simulink model "CP_Gammatone_Filter"  (R2019b)
settings: Solver=VariableStepAuto  StartTime=0.0  StopTime=testtime  RelTol=1e-3
InitFcn:
  | CP_Gammatone_Test_Parameters
StopFcn:
  | Verify_CP_Gammatone_Filter
values from neighbouring files (symbols this model uses):
  cordiciterationswb = 52    [CP_Gammatone_Test_Parameters.m]
  delta_phase = -TWOPI*centerfreq*tdres    [CP_Gammatone_Test_Parameters.m]
  Fs = 48e3    (= 48000)    [CP_Gammatone_Test_Parameters.m]
  tauwb = 0.003    [CP_Gammatone_Test_Parameters.m]
  tdres = 1/Fs    (= 2.08333333333e-05)    [CP_Gammatone_Test_Parameters.m]
  wbgain = 40.766    [CP_Gammatone_Test_Parameters.m]
undefined symbols (not defined in the file or in its folder): jsin
libraries: dspsrcs4 x2
settings Model: Creator=mblun  LastModifiedBy=t96f346
settings SFSimCC: CustomCodeUndefinedFunction=UseInterfaceOnly

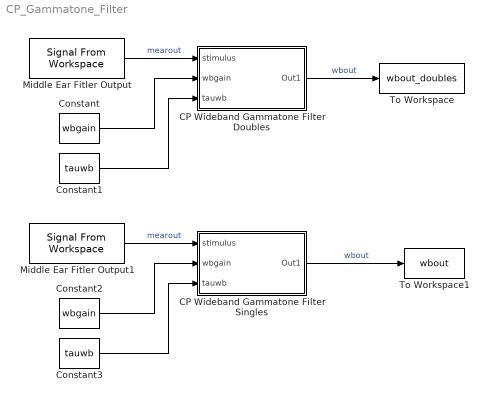
== system CP_Gammatone_Filter ==
  CP Wideband Gammatone Filter Doubles : Subsystem
  CP Wideband Gammatone Filter Singles : Subsystem
  Constant : Constant  Value=wbgain  SampleTime=-1
  Constant1 : Constant  Value=tauwb  SampleTime=-1
  Constant2 : Constant  Value=wbgain  OutDataTypeStr=single  SampleTime=-1
  Constant3 : Constant  Value=tauwb  OutDataTypeStr=single  SampleTime=-1
  Middle Ear Fitler Output : dspsrcs4/Signal From Workspace  X=RxSignal_doubles  Ts=1/Fs  nsamps=1  OutputAfterFinalValue=Setting to zero  ignoreOrWarnInputAndFrameLengths=off  OutputFrames=off
  Middle Ear Fitler Output1 : dspsrcs4/Signal From Workspace  X=RxSignal  Ts=1/Fs  nsamps=1  OutputAfterFinalValue=Setting to zero  ignoreOrWarnInputAndFrameLengths=off  OutputFrames=off
  To Workspace : ToWorkspace  VariableName=wbout_doubles  SampleTime=-1
      settings: Save2DSignal=2-D array (concatenate along first dimension)
  To Workspace1 : ToWorkspace  VariableName=wbout  SampleTime=-1
      settings: Save2DSignal=2-D array (concatenate along first dimension)
  wires:
  Middle Ear Fitler Output/1 -> CP Wideband Gammatone Filter Doubles/1(stimulus)  "mearout"
  CP Wideband Gammatone Filter Doubles/1(Out1) -> To Workspace/1  "wbout"
  Constant/1 -> CP Wideband Gammatone Filter Doubles/2(wbgain)
  Constant1/1 -> CP Wideband Gammatone Filter Doubles/3(tauwb)
  Constant3/1 -> CP Wideband Gammatone Filter Singles/3(tauwb)
  Middle Ear Fitler Output1/1 -> CP Wideband Gammatone Filter Singles/1(stimulus)  "mearout"
  CP Wideband Gammatone Filter Singles/1(Out1) -> To Workspace1/1  "wbout"
  Constant2/1 -> CP Wideband Gammatone Filter Singles/2(wbgain)

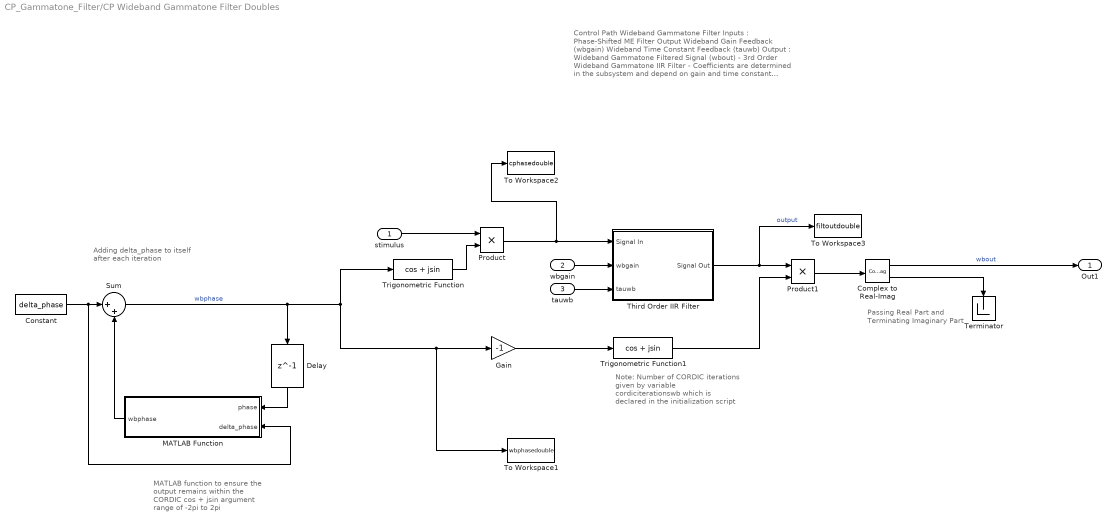
== system CP_Gammatone_Filter/CP Wideband Gammatone Filter Doubles ==
  note: Adding delta_phase to itself after each iteration
  note: Note: Number of CORDIC iterations given by variable cordiciterationswb which is declared in the initialization script
  note: MATLAB function to ensure the output remains within the CORDIC cos + jsin argument range of -2pi to 2pi
  note: Control Path Wideband Gammatone Filter
      |
      | Inputs : Phase-Shifted ME Filter Output
      | Wideband Gain Feedback (wbgain)
      | Wideband Time Constant Feedback (tauwb)
      |
      | Output : Wideband Gammatone Filtered Signal (wbout)
      |
      | - 3rd Order Wideband Gammatone IIR Filter
      |
      | - Coefficients are determined in the subsystem and depend on gain and time constant feedback, set to constants for testing
      |
      | - Implemented w/ Direct Form I Block Structure
  note: Passing Real Part and Terminating Imaginary Part
  stimulus : Inport
  wbgain : Inport  Port=2
  tauwb : Inport  Port=3
  Complex to Real-Imag : ComplexToRealImag
  Constant : Constant  Value=delta_phase  SampleTime=-1
  Delay : Delay  DelayLength=1  InitialCondition=0  UseCircularBuffer=on
  Gain : Gain  Gain=-1
  MATLAB Function : MATLAB Function  TreatAsAtomicUnit=on
  Product : Product
  Product1 : Product
  Sum : Sum  Inputs=|++
  Terminator : Terminator
  Third Order IIR Filter : Subsystem
  To Workspace1 : ToWorkspace  VariableName=wbphasedouble  SampleTime=-1
      settings: Save2DSignal=2-D array (concatenate along first dimension)
  To Workspace2 : ToWorkspace  VariableName=cphasedouble  SampleTime=-1
      settings: Save2DSignal=2-D array (concatenate along first dimension)
  To Workspace3 : ToWorkspace  VariableName=filtoutdouble  SampleTime=-1
      settings: Save2DSignal=2-D array (concatenate along first dimension)
  Trigonometric Function : Trigonometry  Operator=cos + jsin  ApproximationMethod=CORDIC  NumberOfIterations=cordiciterationswb
  Trigonometric Function1 : Trigonometry  Operator=cos + jsin  ApproximationMethod=CORDIC  NumberOfIterations=cordiciterationswb
  Out1 : Outport  VectorParamsAs1DForOutWhenUnconnected=off
  wires:
  wbgain/1 -> Third Order IIR Filter/2(wbgain)
  Gain/1 -> Trigonometric Function1/1
  tauwb/1 -> Third Order IIR Filter/3(tauwb)
  Complex to Real-Imag/2 -> Terminator/1
  Trigonometric Function1/1 -> Product1/2
  Product/1 -> To Workspace2/1, Third Order IIR Filter/1(Signal In)
  Sum/1 -> To Workspace1/1, Gain/1, Trigonometric Function/1, Delay/1  "wbphase"
  Trigonometric Function/1 -> Product/2
  Complex to Real-Imag/1 -> Out1/1  "wbout"
  Constant/1 -> Sum/1, MATLAB Function/2(delta_phase)
  stimulus/1 -> Product/1
  Product1/1 -> Complex to Real-Imag/1
  Third Order IIR Filter/1(Signal Out) -> To Workspace3/1, Product1/1  "output"
  Delay/1 -> MATLAB Function/1(phase)
  MATLAB Function/1(wbphase) -> Sum/2

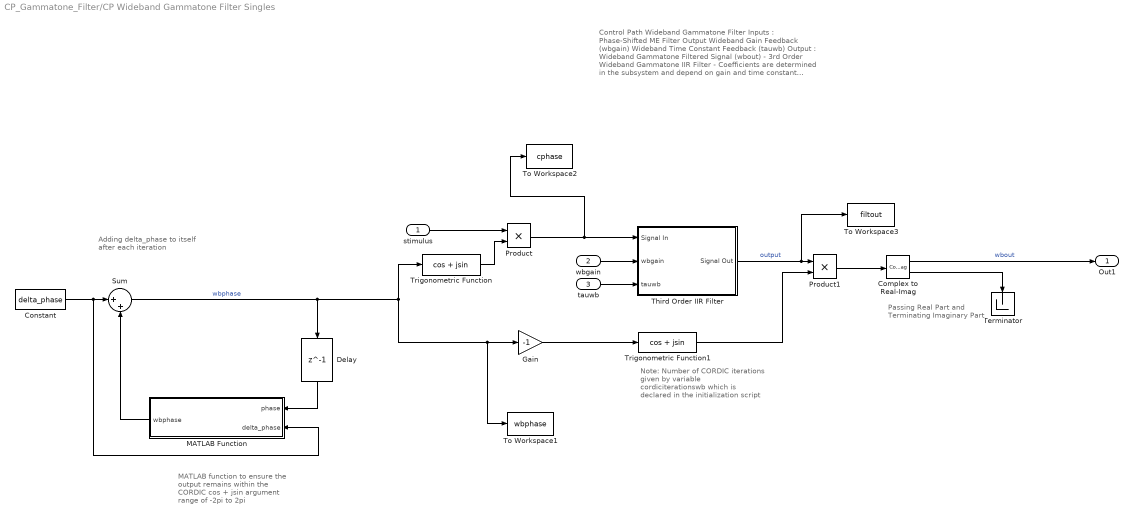
== system CP_Gammatone_Filter/CP Wideband Gammatone Filter Singles ==
  note: Adding delta_phase to itself after each iteration
  note: Note: Number of CORDIC iterations given by variable cordiciterationswb which is declared in the initialization script
  note: MATLAB function to ensure the output remains within the CORDIC cos + jsin argument range of -2pi to 2pi
  note: Control Path Wideband Gammatone Filter
      |
      | Inputs : Phase-Shifted ME Filter Output
      | Wideband Gain Feedback (wbgain)
      | Wideband Time Constant Feedback (tauwb)
      |
      | Output : Wideband Gammatone Filtered Signal (wbout)
      |
      | - 3rd Order Wideband Gammatone IIR Filter
      |
      | - Coefficients are determined in the subsystem and depend on gain and time constant feedback, set to constants for testing
      |
      | - Implemented w/ Direct Form I Block Structure
  note: Passing Real Part and Terminating Imaginary Part
  stimulus : Inport  OutDataTypeStr=single
  wbgain : Inport  Port=2  OutDataTypeStr=single
  tauwb : Inport  Port=3  OutDataTypeStr=single
  Complex to Real-Imag : ComplexToRealImag
  Constant : Constant  Value=delta_phase  OutDataTypeStr=single  SampleTime=-1
  Delay : Delay  DelayLength=1  InitialCondition=0  UseCircularBuffer=on
  Gain : Gain  Gain=-1  OutDataTypeStr=single
  MATLAB Function : MATLAB Function  TreatAsAtomicUnit=on
  Product : Product  OutDataTypeStr=single
  Product1 : Product  OutDataTypeStr=single
  Sum : Sum  Inputs=|++  AccumDataTypeStr=single  OutDataTypeStr=single
  Terminator : Terminator
  Third Order IIR Filter : Subsystem
  To Workspace1 : ToWorkspace  VariableName=wbphase  SampleTime=-1
      settings: Save2DSignal=2-D array (concatenate along first dimension)
  To Workspace2 : ToWorkspace  VariableName=cphase  SampleTime=-1
      settings: Save2DSignal=2-D array (concatenate along first dimension)
  To Workspace3 : ToWorkspace  VariableName=filtout  SampleTime=-1
      settings: Save2DSignal=2-D array (concatenate along first dimension)
  Trigonometric Function : Trigonometry  Operator=cos + jsin  ApproximationMethod=CORDIC  NumberOfIterations=cordiciterationswb
  Trigonometric Function1 : Trigonometry  Operator=cos + jsin  ApproximationMethod=CORDIC  NumberOfIterations=cordiciterationswb
  Out1 : Outport  VectorParamsAs1DForOutWhenUnconnected=off
  wires:
  wbgain/1 -> Third Order IIR Filter/2(wbgain)
  Gain/1 -> Trigonometric Function1/1
  tauwb/1 -> Third Order IIR Filter/3(tauwb)
  Complex to Real-Imag/2 -> Terminator/1
  Trigonometric Function1/1 -> Product1/2
  Product/1 -> To Workspace2/1, Third Order IIR Filter/1(Signal In)
  Sum/1 -> Delay/1, To Workspace1/1, Gain/1, Trigonometric Function/1  "wbphase"
  Trigonometric Function/1 -> Product/2
  Complex to Real-Imag/1 -> Out1/1  "wbout"
  Constant/1 -> Sum/1, MATLAB Function/2(delta_phase)
  stimulus/1 -> Product/1
  Product1/1 -> Complex to Real-Imag/1
  Third Order IIR Filter/1(Signal Out) -> To Workspace3/1, Product1/1  "output"
  Delay/1 -> MATLAB Function/1(phase)
  MATLAB Function/1(wbphase) -> Sum/2

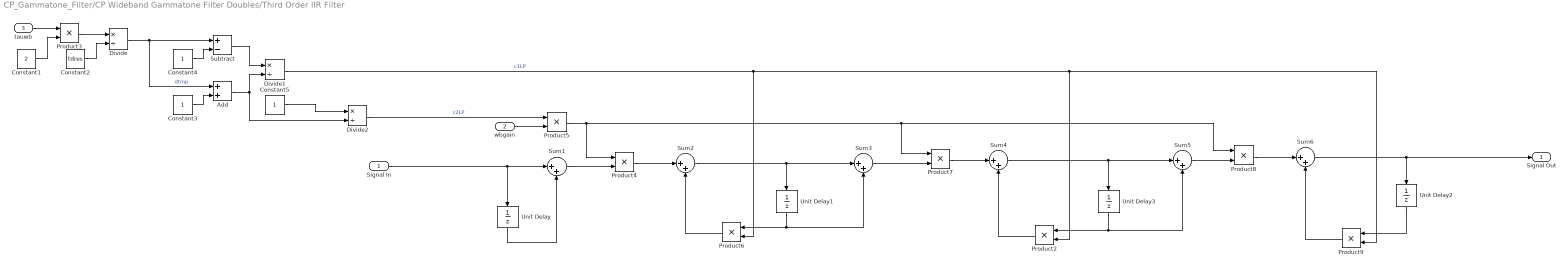
== system CP_Gammatone_Filter/CP Wideband Gammatone Filter Doubles/Third Order IIR Filter ==
  Signal In : Inport
  wbgain : Inport  Port=2
  tauwb : Inport  Port=3
  Add : Sum
  Constant1 : Constant  Value=2  SampleTime=-1
  Constant2 : Constant  Value=tdres  SampleTime=-1
  Constant3 : Constant  SampleTime=-1
  Constant4 : Constant  SampleTime=-1
  Constant5 : Constant  SampleTime=-1
  Divide : Product  Inputs=*/  SaturateOnIntegerOverflow=on  RndMeth=Zero
  Divide1 : Product  Inputs=*/  SaturateOnIntegerOverflow=on  RndMeth=Zero
  Divide2 : Product  Inputs=*/  SaturateOnIntegerOverflow=on  RndMeth=Zero
  Product{2..9} (8 alike) : Product
  Subtract : Sum  Inputs=+-
  Sum{1..6} (6 alike) : Sum  Inputs=|++
  Unit Delay{,1..3} (4 alike) : UnitDelay  SampleTime=-1  HasFrameUpgradeWarning=on
  Signal Out : Outport  VectorParamsAs1DForOutWhenUnconnected=off
  wires:
  Sum6/1 -> Signal Out/1, Unit Delay2/1
  Product8/1 -> Sum6/1
  Subtract/1 -> Divide1/1
  Product2/1 -> Sum4/2
  Signal In/1 -> Unit Delay/1, Sum1/1
  Product5/1 -> Product4/1, Product7/1, Product8/1
  Constant1/1 -> Product3/2
  Divide2/1 -> Product5/1  "c2LP"
  Unit Delay/1 -> Sum1/2
  Divide/1 -> Add/1, Subtract/1  "dtmp"
  Sum3/1 -> Product7/2
  Add/1 -> Divide2/2, Divide1/2
  Sum5/1 -> Product8/2
  Unit Delay1/1 -> Sum3/2, Product6/1
  Constant5/1 -> Divide2/1
  Product7/1 -> Sum4/1
  Product9/1 -> Sum6/2
  Unit Delay3/1 -> Sum5/2, Product2/1
  Sum2/1 -> Sum3/1, Unit Delay1/1
  Product6/1 -> Sum2/2
  Sum4/1 -> Sum5/1, Unit Delay3/1
  tauwb/1 -> Product3/1
  Product3/1 -> Divide/1
  Constant4/1 -> Subtract/2
  wbgain/1 -> Product5/2
  Unit Delay2/1 -> Product9/1
  Product4/1 -> Sum2/1
  Constant2/1 -> Divide/2
  Sum1/1 -> Product4/2
  Constant3/1 -> Add/2
  Divide1/1 -> Product6/2, Product9/2, Product2/2  "c1LP"

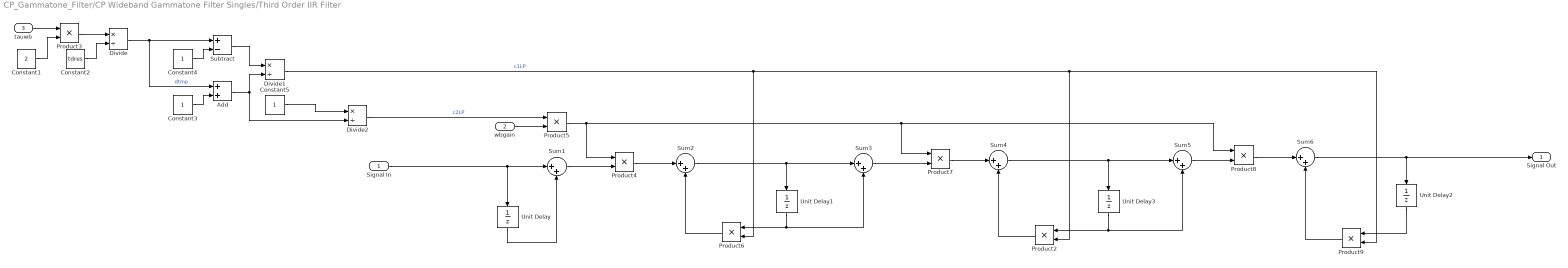
== system CP_Gammatone_Filter/CP Wideband Gammatone Filter Singles/Third Order IIR Filter ==
  Signal In : Inport
  wbgain : Inport  Port=2
  tauwb : Inport  Port=3
  Add : Sum
  Constant1 : Constant  Value=2  OutDataTypeStr=single  SampleTime=-1
  Constant2 : Constant  Value=tdres  OutDataTypeStr=single  SampleTime=-1
  Constant3 : Constant  OutDataTypeStr=single  SampleTime=-1
  Constant4 : Constant  OutDataTypeStr=single  SampleTime=-1
  Constant5 : Constant  OutDataTypeStr=single  SampleTime=-1
  Divide : Product  Inputs=*/  SaturateOnIntegerOverflow=on  RndMeth=Zero
  Divide1 : Product  Inputs=*/  SaturateOnIntegerOverflow=on  RndMeth=Zero
  Divide2 : Product  Inputs=*/  SaturateOnIntegerOverflow=on  RndMeth=Zero
  Product{2..9} (8 alike) : Product
  Subtract : Sum  Inputs=+-
  Sum{1..6} (6 alike) : Sum  Inputs=|++
  Unit Delay{,1..3} (4 alike) : UnitDelay  SampleTime=-1  HasFrameUpgradeWarning=on
  Signal Out : Outport  VectorParamsAs1DForOutWhenUnconnected=off
  wires:
  Sum6/1 -> Signal Out/1, Unit Delay2/1
  Product8/1 -> Sum6/1
  Subtract/1 -> Divide1/1
  Product2/1 -> Sum4/2
  Signal In/1 -> Unit Delay/1, Sum1/1
  Product5/1 -> Product4/1, Product7/1, Product8/1
  Constant1/1 -> Product3/2
  Divide2/1 -> Product5/1  "c2LP"
  Unit Delay/1 -> Sum1/2
  Divide/1 -> Add/1, Subtract/1  "dtmp"
  Sum3/1 -> Product7/2
  Add/1 -> Divide2/2, Divide1/2
  Sum5/1 -> Product8/2
  Unit Delay1/1 -> Sum3/2, Product6/1
  Constant5/1 -> Divide2/1
  Product7/1 -> Sum4/1
  Product9/1 -> Sum6/2
  Unit Delay3/1 -> Sum5/2, Product2/1
  Sum2/1 -> Sum3/1, Unit Delay1/1
  Product6/1 -> Sum2/2
  Sum4/1 -> Sum5/1, Unit Delay3/1
  tauwb/1 -> Product3/1
  Product3/1 -> Divide/1
  Constant4/1 -> Subtract/2
  wbgain/1 -> Product5/2
  Unit Delay2/1 -> Product9/1
  Product4/1 -> Sum2/1
  Constant2/1 -> Divide/2
  Sum1/1 -> Product4/2
  Constant3/1 -> Add/2
  Divide1/1 -> Product6/2, Product9/2, Product2/2  "c1LP"

== matlab function CP_Gammatone_Filter/CP Wideband Gammatone Filter Singles/MATLAB Function ==
  data: phase input; wbphase output; delta_phase input
% Matthew Blunt
% Speech % Hearing Internship
% Check Gammatone Cosine Argument
% 6/6/2019

% ---------------------------------------------------------------------- %
% NOTES: 
% ---------------------------------------------------------------------- %

% The following script is designed to work within the CP Wideband Gammatone
% Filter Simulink model in order to ensure that the argument of the
% trigonometric representation of a complex exponential remains within
% [-2pi,2pi). The function will simply take in the wb phase variable and
% output the same value in radians that falls within the range of arguments
% for the Simulink trigonometric block.

% *** NOTE: Edited by Matthew Blunt 03/05/2020
% *** Now evaluates bounds in the feedback loop to ensure stability for
% FPGA implementation

% ---------------------------------------------------------------------- %
% CODE: 
% ---------------------------------------------------------------------- %

% *** Edited by Matthew Blunt 03/05/2020
% *** Only accounts for negative values of delta_phase
function wbphase = WbGammaToneCosineArgCheck(phase,delta_phase)
    if phase <= (-2*pi - delta_phase)
        phase = phase+2*pi;
    end
    wbphase = phase;
end

== matlab function CP_Gammatone_Filter/CP Wideband Gammatone Filter Doubles/MATLAB Function ==
  data: phase input; wbphase output; delta_phase input
% Matthew Blunt
% Speech % Hearing Internship
% Check Gammatone Cosine Argument
% 6/6/2019

% ---------------------------------------------------------------------- %
% NOTES: 
% ---------------------------------------------------------------------- %

% The following script is designed to work within the CP Wideband Gammatone
% Filter Simulink model in order to ensure that the argument of the
% trigonometric representation of a complex exponential remains within
% [-2pi,2pi). The function will simply take in the wb phase variable and
% output the same value in radians that falls within the range of arguments
% for the Simulink trigonometric block.

% *** NOTE: Edited by Matthew Blunt 03/05/2020
% *** Now evaluates bounds in the feedback loop to ensure stability for
% FPGA implementation

% ---------------------------------------------------------------------- %
% CODE: 
% ---------------------------------------------------------------------- %

% *** Edited by Matthew Blunt 03/05/2020
% *** Only accounts for negative values of delta_phase
function wbphase = WbGammaToneCosineArgCheck(phase,delta_phase)
    if phase <= (-2*pi - delta_phase)
        phase = phase+2*pi;
    end
    wbphase = phase;
end
